simulink model "pmsm_mpc_ekf"  (R2022a)
settings: Solver=ode23tb  StartTime=0.0  StopTime=simlength  FixedStep=tsample  MaxStep=ts
values from neighbouring files (symbols this model uses):
  ki_w = 1    [init.m]    (also in init_2022_05_28.m)
  kp_w = 2    [init.m]    (also in init_2022_05_28.m)
  simlength = 60    [init.m]    (also in init_2022_05_28.m)
  tcontrol = 1/fPWM_INV/6    (= 2.08333333333e-05)    [init.m]    (also in init_2022_05_28.m)
  ts = tcontrol    (= 2.08333333333e-05)    [init.m]    (also in init_2022_05_28.m)
undefined symbols (not defined in the file or in its folder): A1_tilde, A2_tilde, A3_tilde, A4_tilde, Adrso, b, b_brake, Bd, C, Crso, ibez, Jm, Lalpha, Lbeta, Ldrso, omega_bez, omega_m_bez, omega_m_sim, psi_m, Qkalman, Rkalman, Rs, tau_bez, Vdc
libraries: nesl_utility x14, fl_lib x7, pmsm_alphabeta_lib x1
settings Model: SimulationMode=accelerator  Creator=dbagn  LastModifiedBy=dabagnara
settings SolverCC: NumberNewtonIterations=3  ZeroCrossControl=DisableAll  AlgebraicLoopSolver=TrustRegion  SolverResetMethod=Robust
settings DataIOCC: ReturnWorkspaceOutputs=off
settings DebuggingCC: UnconnectedInputMsg=warning  UnconnectedOutputMsg=warning  UnconnectedLineMsg=warning  SFMachineParentedDataDiag=warning
settings RTWCC: DLArmComputeVersion=19.05

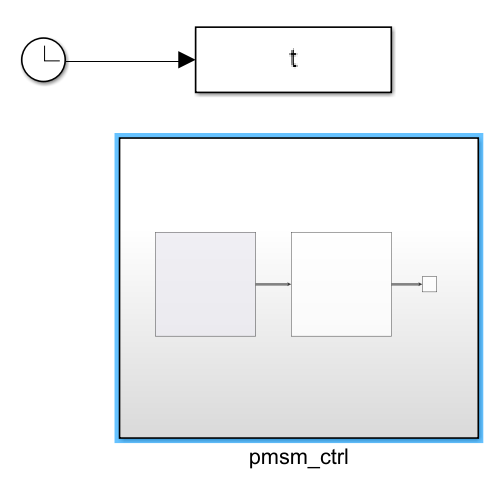
[thumbnail: Simulink's stored preview of the top-level diagram]
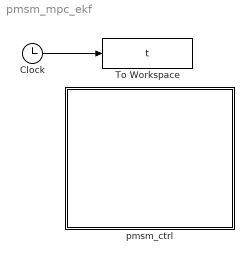
== system pmsm_mpc_ekf ==
  Clock : Clock
  To Workspace : ToWorkspace  VariableName=t  SampleTime=ts
      settings: MaxDataPoints=Nc
  pmsm_ctrl : Subsystem
  wires:
  Clock/1 -> To Workspace/1

== system pmsm_mpc_ekf/pmsm_ctrl ==
  pmsm : Subsystem
  pmsm_control : Subsystem
  pmsm_data : Scope
  wires:
  pmsm_control/1(ualphabeta) -> pmsm/1(u_alphabeta)
  pmsm/1(pmsm_data) -> pmsm_data/1

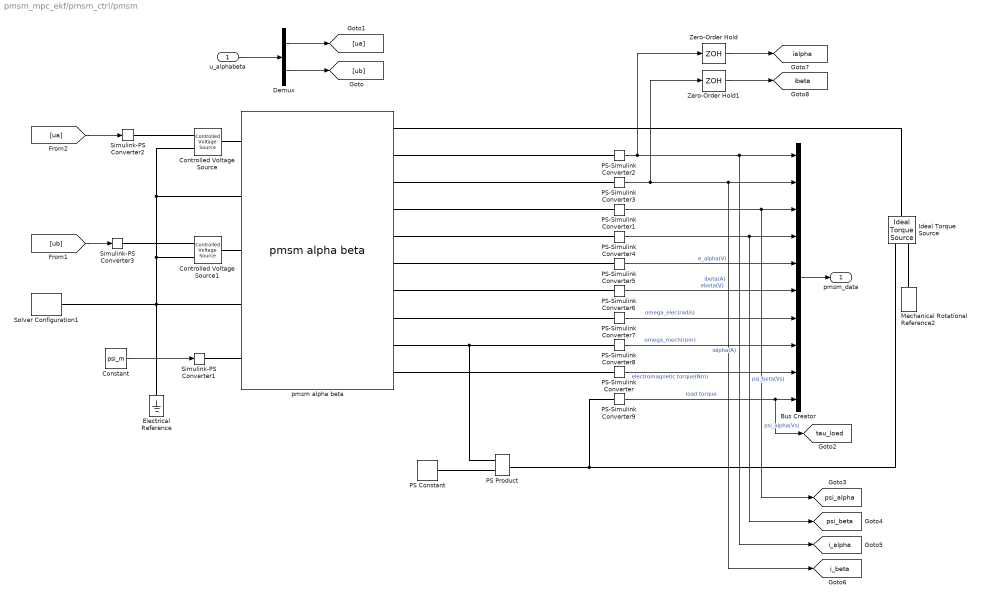
== system pmsm_mpc_ekf/pmsm_ctrl/pmsm ==
  u_alphabeta : Inport
  Bus Creator : BusCreator  Inputs=10
  Constant : Constant  Value=psi_m
  Controlled Voltage Source : fl_lib/Electrical/Electrical Sources/Controlled Voltage Source
      settings: SourceProductBaseCode=PW,SS,VE
  Controlled Voltage Source1 : fl_lib/Electrical/Electrical Sources/Controlled Voltage Source
      settings: SourceProductBaseCode=PW,SS,VE
  Demux : Demux  Outputs=2
  Electrical Reference : fl_lib/Electrical/Electrical Elements/Electrical Reference
      settings: SourceProductBaseCode=PW,SS,VE
  Ideal Torque Source : fl_lib/Mechanical/Mechanical Sources/Ideal Torque Source
      settings: SourceProductBaseCode=PW,SS,VE
  Mechanical Rotational Reference2 : fl_lib/Mechanical/Rotational Elements/Mechanical Rotational Reference
      settings: SourceProductBaseCode=PW,SS,VE
  PS Constant : fl_lib/Physical Signals/Sources/PS Constant  constant=-b_brake N*m/(rad/s)
      settings: SourceProductBaseCode=PW,SS,VE
  PS Product : fl_lib/Physical Signals/Functions/PS Product
      settings: SourceProductBaseCode=PW,SS,VE
  PS-Simulink Converter : nesl_utility/PS-Simulink Converter  PhysicalDomain=network_engine_domain  SubClassName=ps_output  LeftPortType=input  RightPortType=output  PseudoPeriodic=off  Frequencies=[]  VectorFormat=1-D array  Unit=N*m  AffineConversion=on
      settings: SourceProductBaseCode=SS,PW,VE
  PS-Simulink Converter1 : nesl_utility/PS-Simulink Converter  PhysicalDomain=network_engine_domain  SubClassName=ps_output  LeftPortType=input  RightPortType=output  PseudoPeriodic=off  Frequencies=[]  VectorFormat=1-D array  Unit=V*s  AffineConversion=on
      settings: SourceProductBaseCode=SS,PW,VE
  PS-Simulink Converter2 : nesl_utility/PS-Simulink Converter  PhysicalDomain=network_engine_domain  SubClassName=ps_output  LeftPortType=input  RightPortType=output  PseudoPeriodic=off  Frequencies=[]  VectorFormat=1-D array  Unit=A  AffineConversion=on
      settings: SourceProductBaseCode=SS,PW,VE
  PS-Simulink Converter3 : nesl_utility/PS-Simulink Converter  PhysicalDomain=network_engine_domain  SubClassName=ps_output  LeftPortType=input  RightPortType=output  PseudoPeriodic=off  Frequencies=[]  VectorFormat=1-D array  Unit=A  AffineConversion=on
      settings: SourceProductBaseCode=SS,PW,VE
  PS-Simulink Converter4 : nesl_utility/PS-Simulink Converter  PhysicalDomain=network_engine_domain  SubClassName=ps_output  LeftPortType=input  RightPortType=output  PseudoPeriodic=off  Frequencies=[]  VectorFormat=1-D array  Unit=V*s  AffineConversion=on
      settings: SourceProductBaseCode=SS,PW,VE
  PS-Simulink Converter5 : nesl_utility/PS-Simulink Converter  PhysicalDomain=network_engine_domain  SubClassName=ps_output  LeftPortType=input  RightPortType=output  PseudoPeriodic=off  Frequencies=[]  VectorFormat=1-D array  Unit=V  AffineConversion=on
      settings: SourceProductBaseCode=SS,PW,VE
  PS-Simulink Converter6 : nesl_utility/PS-Simulink Converter  PhysicalDomain=network_engine_domain  SubClassName=ps_output  LeftPortType=input  RightPortType=output  PseudoPeriodic=off  Frequencies=[]  VectorFormat=1-D array  Unit=V  AffineConversion=on
      settings: SourceProductBaseCode=SS,PW,VE
  PS-Simulink Converter7 : nesl_utility/PS-Simulink Converter  PhysicalDomain=network_engine_domain  SubClassName=ps_output  LeftPortType=input  RightPortType=output  PseudoPeriodic=off  Frequencies=[]  VectorFormat=1-D array  Unit=rad/s  AffineConversion=on
      settings: SourceProductBaseCode=SS,PW,VE
  PS-Simulink Converter8 : nesl_utility/PS-Simulink Converter  PhysicalDomain=network_engine_domain  SubClassName=ps_output  LeftPortType=input  RightPortType=output  PseudoPeriodic=off  Frequencies=[]  VectorFormat=1-D array  Unit=rpm  AffineConversion=on
      settings: SourceProductBaseCode=SS,PW,VE
  PS-Simulink Converter9 : nesl_utility/PS-Simulink Converter  PhysicalDomain=network_engine_domain  SubClassName=ps_output  LeftPortType=input  RightPortType=output  PseudoPeriodic=off  Frequencies=[]  VectorFormat=1-D array  Unit=N*m  AffineConversion=on
      settings: SourceProductBaseCode=SS,PW,VE
  Simulink-PS Converter1 : nesl_utility/Simulink-PS Converter  PhysicalDomain=network_engine_domain  SubClassName=ps_input  LeftPortType=input  RightPortType=output  PseudoPeriodic=off  Frequencies=[]  NoiseDistribution=none  NoiseParameters=[]  Unit=V*s  AffineConversion=off  FilteringAndDerivatives=provide  SimscapeFilterOrder=1  InputFilterTimeConstant=0.001  UdotUserProvided=0
      settings: SourceProductBaseCode=SS,PW,VE
  Simulink-PS Converter2 : nesl_utility/Simulink-PS Converter  PhysicalDomain=network_engine_domain  SubClassName=ps_input  LeftPortType=input  RightPortType=output  PseudoPeriodic=off  Frequencies=[]  NoiseDistribution=none  NoiseParameters=[]  Unit=1  AffineConversion=off  FilteringAndDerivatives=provide  SimscapeFilterOrder=1  InputFilterTimeConstant=0.001  UdotUserProvided=0
      settings: SourceProductBaseCode=SS,PW,VE
  Simulink-PS Converter3 : nesl_utility/Simulink-PS Converter  PhysicalDomain=network_engine_domain  SubClassName=ps_input  LeftPortType=input  RightPortType=output  PseudoPeriodic=off  Frequencies=[]  NoiseDistribution=none  NoiseParameters=[]  Unit=1  AffineConversion=off  FilteringAndDerivatives=provide  SimscapeFilterOrder=1  InputFilterTimeConstant=0.001  UdotUserProvided=0
      settings: SourceProductBaseCode=SS,PW,VE
  Solver Configuration1 : nesl_utility/Solver Configuration  PhysicalDomain=network_engine_domain  SubClassName=solver  LeftPortType=input  RightPortType=generic  Tones=[]  Harmonics=[]  SimulateNoise=off  Profile=off  UseLocalSampling=off  EnableSwitchedLinearOptims=on  FrequencyDomain=off  UseCCode=off  RelTol=0.001  AbsTol=1e-06  MinStep=1e-09  ToWorkspace=off  RevertToSquareIcSolve=off  NumHomotopyIterations=100  PhasorMode=off  PhasorModeNumHarmonics=1  IndexReductionMethod=DerivativeReplacement  DoDC=on  ResidualTolerance=1e-09  UseLocalSolver=on  LocalSolverChoice=NE_TRAPEZOIDAL_ADVANCER  LocalSolverSampleTime=ts  DoFixedCost=on  MaxNonlinIter=3  MaxModeIter=2  ComputeImpulses=off  ImpulseIterations=2  LinearAlgebra=auto  LinearAlgebraNumThread=0  EquationFormulation=NE_TIME_EF  DelaysMemoryBudget=1024*4  AutomaticFiltering=on  FilteringTimeConstant=ts  PartitionStorageMethod=AS_NEEDED  PartitionMemoryBudget=1024  PartitionMethod=ROBUST
      settings: SourceProductBaseCode=SS,PW,VE
  Zero-Order Hold : ZeroOrderHold  SampleTime=tcontrol
  Zero-Order Hold1 : ZeroOrderHold  SampleTime=tcontrol
  pmsm alpha beta : pmsm_alphabeta_lib/pmsm alpha beta  number_poles=number_poles  Lalpha=Lalpha H  Lbeta=Lbeta H  Rs=Rs Ohm  J=Jm kg*m^2  b=b N*m/(rad/s)  theta_specify=off  theta_priority=None  theta=0 rad  theta_nominal_specify=off  theta_nominal_unit=rad  theta_nominal_value=1  omega_specify=off  omega_priority=None  omega=0 rad/s  omega_nominal_specify=off  omega_nominal_unit=rad/s  omega_nominal_value=1  omega_m_specify=off  omega_m_priority=None  omega_m=0 rad/s  omega_m_nominal_specify=off  omega_m_nominal_unit=rad/s  omega_m_nominal_value=1  ialpha_specify=on  ialpha_priority=High  ialpha=0 A  ialpha_nominal_specify=off  ialpha_nominal_unit=A  ialpha_nominal_value=1  ibeta_specify=on  ibeta_priority=High  ibeta=0 A  ibeta_nominal_specify=off  ibeta_nominal_unit=A  ibeta_nominal_value=1  psi_alpha_specify=off  psi_alpha_priority=None  psi_alpha=0 V*s  psi_alpha_nominal_specify=off  psi_alpha_nominal_unit=V*s  psi_alpha_nominal_value=1  psi_beta_specify=off  psi_beta_priority=High  psi_beta=0.0 V*s  psi_beta_nominal_specify=off  psi_beta_nominal_unit=V*s  psi_beta_nominal_value=1  ualpha_specify=off  ualpha_priority=None  ualpha=0 V  ualpha_nominal_specify=off  ualpha_nominal_unit=V  ualpha_nominal_value=1  ubeta_specify=off  ubeta_priority=None  ubeta=0 V  ubeta_nominal_specify=off  ubeta_nominal_unit=V  ubeta_nominal_value=1  tau_load_specify=off  tau_load_priority=None  tau_load=0 N*m  tau_load_nominal_specify=off  tau_load_nominal_unit=N*m  tau_load_nominal_value=1
      settings: InternalSimscapePortConfiguration="{\"Bottom\":[],\"Left\":[{\"id\":\"u_alpha_p\",\"label\":\"_u_alpha+_\",\"type\":\"foundation.electrical.electrical\"},{\"id\":\"u_alpha_n\",\"label\":\"_u_alpha-_\",\"type\":\"foundation.electrical.electrical\"},{\"id\":\"u_beta_p\",\"label\":\"_u_beta+_\",\"type\":\"foundation.electrical.electrical\"},{\"id\":\"u_beta_n\",\"label\":\"_u_beta-_\",\"type\":\"foundation.electrical.electrical\"},{\"id\":\"psi_m\",\"label\":\"_psi_m_\",\"type\":\"input\"}],\"Right\":[{\"id\":\"s\",\"label\":\"_s_\",\"type\":\"foundation.mechanical.rotational.rotational\"},{\"id\":\"i_alpha_out\",\"label\":\"_i_alpha_\",\"type\":\"output\"},{\"id\":\"i_beta_out\",\"label\":\"_i_beta_\",\"type\":\"output\"},{\"id\":\"psi_alpha_out\",\"label\":\"_psi_alpha_\",\"type\":\"output\"},{\"id\":\"psi_beta_out\",\"label\":\"_psi_beta_\",\"type\":\"output\"},{\"id\":\"e_alpha_out\",\"label\":\"_e_alpha_\",\"type\":\"output\"},{\"id\":\"e_beta_out\",\"label\":\"_e_beta_\",\"type\":\"output\"},{\"id\":\"omega_elec_out\",\"label\":\"_omega_elec_\",\"type\":\"output\"},{\"id\":\"omega_mech_out\",\"label\":\"_omega_mech_\",\"type\":\"output\"},{\"id\":\"torque_e_out\",\"label\":\"_torque_e_\",\"type\":\"output\"}],\"Top\":[]}"
  pmsm_data : Outport
  tag scope: i_alpha=global, i_beta=global, ialpha=global, ibeta=global, psi_alpha=global, psi_beta=global, tau_load=global
  wires:
  [ua] -> Simulink-PS Converter2/1
  [ub] -> Simulink-PS Converter3/1
  u_alphabeta/1 -> Demux/1
  Demux/1 -> [ua]
  Demux/2 -> [ub]
  Zero-Order Hold/1 -> [ialpha]
  Zero-Order Hold1/1 -> [ibeta]
  PS-Simulink Converter2/1 -> [i_alpha], Bus Creator/1, Zero-Order Hold/1  "ialpha(A)"
  PS-Simulink Converter3/1 -> [i_beta], Bus Creator/2, Zero-Order Hold1/1  "ibeta(A)"
  PS-Simulink Converter1/1 -> [psi_alpha], Bus Creator/3  "psi_alpha(Vs)"
  PS-Simulink Converter4/1 -> Bus Creator/4, [psi_beta]  "psi_beta(Vs)"
  PS-Simulink Converter5/1 -> Bus Creator/5  "e_alpha(V)"
  PS-Simulink Converter6/1 -> Bus Creator/6  "ebeta(V)"
  PS-Simulink Converter7/1 -> Bus Creator/7  "omega_elec(rad/s)"
  PS-Simulink Converter8/1 -> Bus Creator/8  "omega_mech(rpm)"
  PS-Simulink Converter/1 -> Bus Creator/9  "electromagnetic torque(Nm)"
  PS-Simulink Converter9/1 -> Bus Creator/10, [tau_load]  "load torque"
  Bus Creator/1 -> pmsm_data/1
  Constant/1 -> Simulink-PS Converter1/1
  connections:
  Controlled Voltage Source/RConn1 -- Simulink-PS Converter2/RConn1
  pmsm alpha beta/LConn1 -- Controlled Voltage Source/LConn1
  Simulink-PS Converter3/RConn1 -- Controlled Voltage Source1/RConn1
  pmsm alpha beta/LConn3 -- Controlled Voltage Source1/LConn1
  Controlled Voltage Source/RConn2 -- Controlled Voltage Source1/RConn2 -- pmsm alpha beta/LConn4 -- Electrical Reference/LConn1 -- Solver Configuration1/RConn1 -- pmsm alpha beta/LConn2
  pmsm alpha beta/RConn2 -- PS-Simulink Converter2/LConn1
  pmsm alpha beta/RConn3 -- PS-Simulink Converter3/LConn1
  PS-Simulink Converter4/LConn1 -- pmsm alpha beta/RConn5
  PS-Simulink Converter1/LConn1 -- pmsm alpha beta/RConn4
  PS-Simulink Converter5/LConn1 -- pmsm alpha beta/RConn6
  pmsm alpha beta/RConn7 -- PS-Simulink Converter6/LConn1
  Mechanical Rotational Reference2/LConn1 -- Ideal Torque Source/RConn2
  pmsm alpha beta/RConn1 -- Ideal Torque Source/LConn1
  pmsm alpha beta/RConn9 -- PS-Simulink Converter8/LConn1 -- PS Product/LConn1
  pmsm alpha beta/RConn10 -- PS-Simulink Converter/LConn1
  PS Constant/RConn1 -- PS Product/LConn2
  PS Product/RConn1 -- Ideal Torque Source/RConn1 -- PS-Simulink Converter9/LConn1
  pmsm alpha beta/RConn8 -- PS-Simulink Converter7/LConn1
  Simulink-PS Converter1/RConn1 -- pmsm alpha beta/LConn5

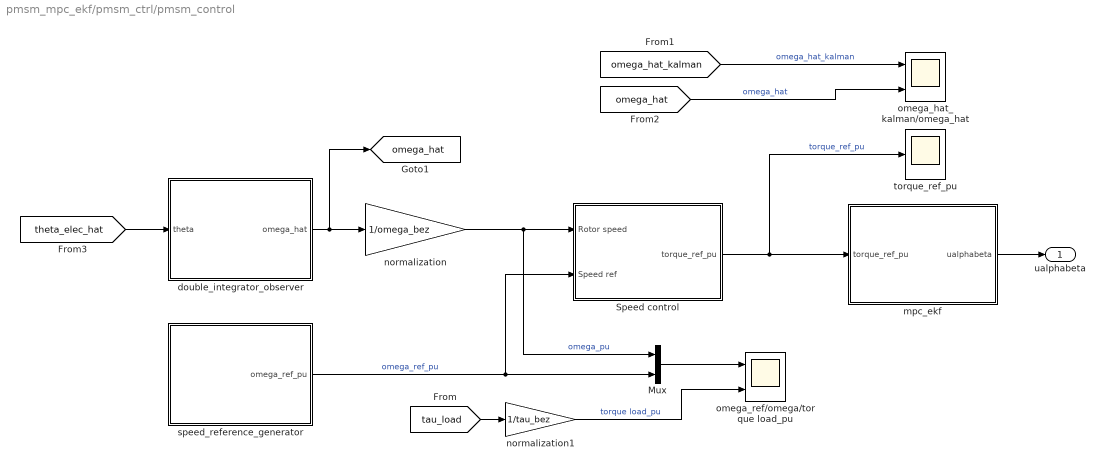
== system pmsm_mpc_ekf/pmsm_ctrl/pmsm_control ==
  Mux : Mux  Inputs=2
  Speed control : Subsystem
  double_integrator_observer : Subsystem
  mpc_ekf : Subsystem
  normalization : Gain  Gain=1/omega_bez
  normalization1 : Gain  Gain=1/tau_bez
  omega_hat_kalman/omega_hat : Scope  NumInputPorts=2
  omega_ref/omega/torque load_pu : Scope  NumInputPorts=2
  speed_reference_generator : Subsystem
  torque_ref_pu : Scope
  ualphabeta : Outport  VectorParamsAs1DForOutWhenUnconnected=off
  tag scope: omega_hat=global
  wires:
  mpc_ekf/1(ualphabeta) -> ualphabeta/1
  normalization/1 -> Mux/1, Speed control/1(Rotor speed)  "omega_pu"
  [theta_elec_hat] -> double_integrator_observer/1(theta)
  Speed control/1(torque_ref_pu) -> torque_ref_pu/1, mpc_ekf/1(torque_ref_pu)  "torque_ref_pu"
  speed_reference_generator/1(omega_ref_pu) -> Speed control/2(Speed ref), Mux/2  "omega_ref_pu"
  Mux/1 -> omega_ref/omega/torque load_pu/1
  [tau_load] -> normalization1/1
  normalization1/1 -> omega_ref/omega/torque load_pu/2  "torque load_pu"
  double_integrator_observer/1(omega_hat) -> [omega_hat], normalization/1
  [omega_hat_kalman] -> omega_hat_kalman/omega_hat/1  "omega_hat_kalman"
  [omega_hat] -> omega_hat_kalman/omega_hat/2  "omega_hat"

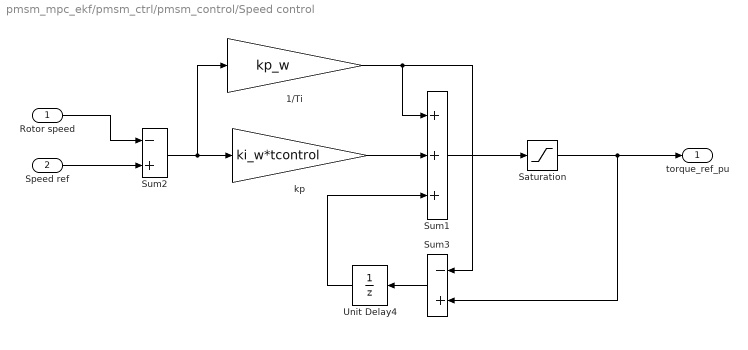
== system pmsm_mpc_ekf/pmsm_ctrl/pmsm_control/Speed control ==
  Rotor speed : Inport
  Speed ref : Inport  Port=2
  1/Ti : Gain  Gain=kp_w  SaturateOnIntegerOverflow=on  OutDataTypeStr=Inherit: Same as input  ParamDataTypeStr=Inherit: Same as input
  Saturation : Saturate  UpperLimit=1.5  LowerLimit=-1.5
  Sum1 : Sum  Inputs=+++  SaturateOnIntegerOverflow=on
  Sum2 : Sum  Inputs=-+  SaturateOnIntegerOverflow=on
  Sum3 : Sum  Inputs=-+  SaturateOnIntegerOverflow=on
  Unit Delay4 : UnitDelay  SampleTime=tcontrol  HasFrameUpgradeWarning=on
  kp : Gain  Gain=ki_w*tcontrol  SaturateOnIntegerOverflow=on  OutDataTypeStr=Inherit: Same as input  ParamDataTypeStr=Inherit: Same as input
  torque_ref_pu : Outport
  wires:
  1/Ti/1 -> Sum1/1, Sum3/1
  kp/1 -> Sum1/2
  Sum3/1 -> Unit Delay4/1
  Unit Delay4/1 -> Sum1/3
  Speed ref/1 -> Sum2/2
  Rotor speed/1 -> Sum2/1
  Sum2/1 -> kp/1, 1/Ti/1
  Saturation/1 -> torque_ref_pu/1, Sum3/2
  Sum1/1 -> Saturation/1

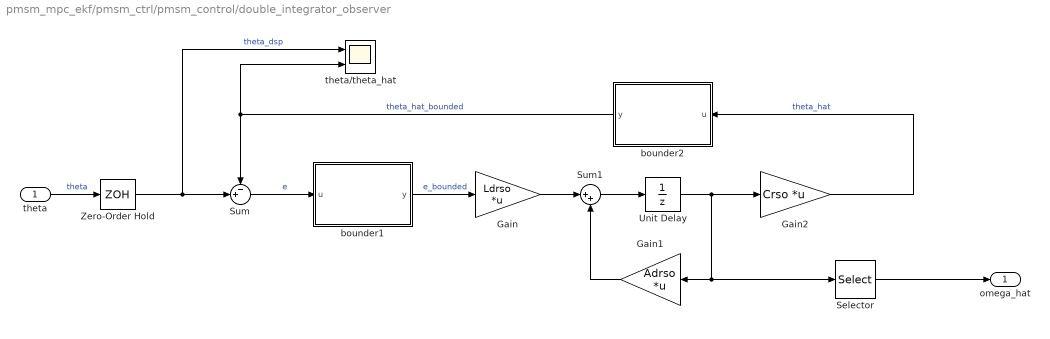
== system pmsm_mpc_ekf/pmsm_ctrl/pmsm_control/double_integrator_observer ==
  theta : Inport
  Gain : Gain  Gain=Ldrso  Multiplication=Matrix(K*u)
  Gain1 : Gain  Gain=Adrso  Multiplication=Matrix(K*u)
  Gain2 : Gain  Gain=Crso  Multiplication=Matrix(K*u)
  Selector : Selector  InputPortWidth=2  IndexOptions=Index vector (dialog)  Indices=2  OutputSizes=1
  Sum : Sum  Inputs=-+|
  Sum1 : Sum  Inputs=|++
  Unit Delay : UnitDelay  SampleTime=tcontrol  HasFrameUpgradeWarning=on
  Zero-Order Hold : ZeroOrderHold  SampleTime=tcontrol
  bounder1 : MATLAB Function  TreatAsAtomicUnit=on  SystemSampleTime=tcontrol
  bounder2 : MATLAB Function  TreatAsAtomicUnit=on  SystemSampleTime=tcontrol
  theta/theta_hat : Scope  NumInputPorts=2
  omega_hat : Outport
  wires:
  Gain/1 -> Sum1/1
  Selector/1 -> omega_hat/1
  Gain2/1 -> bounder2/1(u)  "theta_hat"
  Gain1/1 -> Sum1/2
  Sum1/1 -> Unit Delay/1
  Sum/1 -> bounder1/1(u)  "e"
  Unit Delay/1 -> Gain1/1, Selector/1, Gain2/1
  theta/1 -> Zero-Order Hold/1  "theta"
  Zero-Order Hold/1 -> theta/theta_hat/1, Sum/2  "theta_dsp"
  bounder1/1(y) -> Gain/1  "e_bounded"
  bounder2/1(y) -> theta/theta_hat/2, Sum/1  "theta_hat_bounded"

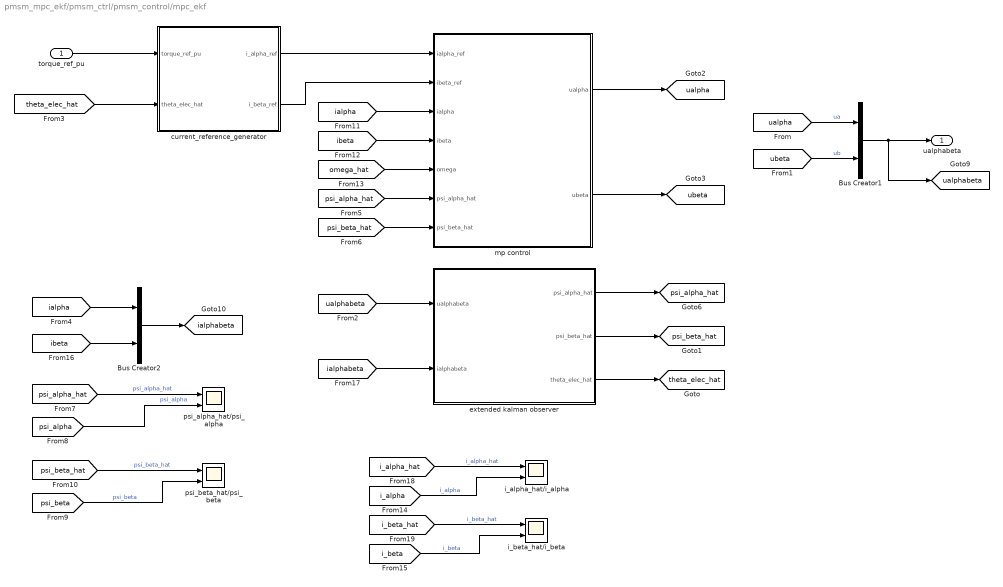
== system pmsm_mpc_ekf/pmsm_ctrl/pmsm_control/mpc_ekf ==
  torque_ref_pu : Inport
  Bus Creator1 : BusCreator  Inputs=2
  Bus Creator2 : BusCreator  Inputs=2
  current_reference_generator : Subsystem
  extended kalman observer : Subsystem
  i_alpha_hat/i_alpha : Scope  NumInputPorts=2
  i_beta_hat/i_beta : Scope  NumInputPorts=2
  mp control : Subsystem
  psi_alpha_hat/psi_alpha : Scope  NumInputPorts=2
  psi_beta_hat/psi_beta : Scope  NumInputPorts=2
  ualphabeta : Outport  VectorParamsAs1DForOutWhenUnconnected=off
  tag scope: ialphabeta=global, psi_alpha_hat=global, psi_beta_hat=global, theta_elec_hat=global, ualpha=global, ualphabeta=global, ubeta=global
  wires:
  [ubeta] -> Bus Creator1/2  "ub"
  [ualpha] -> Bus Creator1/1  "ua"
  Bus Creator1/1 -> [ualphabeta], ualphabeta/1
  torque_ref_pu/1 -> current_reference_generator/1(torque_ref_pu)
  mp control/2(ubeta) -> [ubeta]
  mp control/1(ualpha) -> [ualpha]
  extended kalman observer/1(psi_alpha_hat) -> [psi_alpha_hat]
  extended kalman observer/2(psi_beta_hat) -> [psi_beta_hat]
  [psi_alpha_hat] -> mp control/6(psi_alpha_hat)
  [psi_beta_hat] -> mp control/7(psi_beta_hat)
  [ialpha] -> mp control/3(ialpha)
  [ibeta] -> mp control/4(ibeta)
  [omega_hat] -> mp control/5(omega)
  current_reference_generator/1(i_alpha_ref) -> mp control/1(ialpha_ref)
  current_reference_generator/2(i_beta_ref) -> mp control/2(ibeta_ref)
  [ualphabeta] -> extended kalman observer/1(ualphabeta)
  [ialpha] -> Bus Creator2/1
  [ibeta] -> Bus Creator2/2
  Bus Creator2/1 -> [ialphabeta]
  [ialphabeta] -> extended kalman observer/2(ialphabeta)
  [theta_elec_hat] -> current_reference_generator/2(theta_elec_hat)
  extended kalman observer/3(theta_elec_hat) -> [theta_elec_hat]
  [psi_alpha_hat] -> psi_alpha_hat/psi_alpha/1  "psi_alpha_hat"
  [psi_alpha] -> psi_alpha_hat/psi_alpha/2  "psi_alpha"
  [psi_beta_hat] -> psi_beta_hat/psi_beta/1  "psi_beta_hat"
  [psi_beta] -> psi_beta_hat/psi_beta/2  "psi_beta"
  [i_alpha_hat] -> i_alpha_hat/i_alpha/1  "i_alpha_hat"
  [i_alpha] -> i_alpha_hat/i_alpha/2  "i_alpha"
  [i_beta_hat] -> i_beta_hat/i_beta/1  "i_beta_hat"
  [i_beta] -> i_beta_hat/i_beta/2  "i_beta"

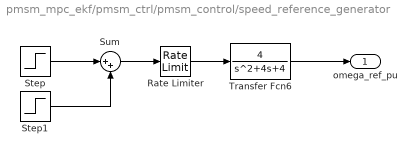
== system pmsm_mpc_ekf/pmsm_ctrl/pmsm_control/speed_reference_generator ==
  Rate Limiter : RateLimiter  RisingSlewLimit=0.25  FallingSlewLimit=-0.25  SampleTimeMode=inherited
  Step : Step  Time=simlength/20  After=omega_m_sim/omega_m_bez  SampleTime=0
  Step1 : Step  Time=simlength/2  After=-2*omega_m_sim/omega_m_bez  SampleTime=0
  Sum : Sum  Inputs=|++
  Transfer Fcn6 : TransferFcn  Numerator=[4]  Denominator=[1 4 4]
  omega_ref_pu : Outport
  wires:
  Rate Limiter/1 -> Transfer Fcn6/1
  Step/1 -> Sum/1
  Transfer Fcn6/1 -> omega_ref_pu/1
  Sum/1 -> Rate Limiter/1
  Step1/1 -> Sum/2

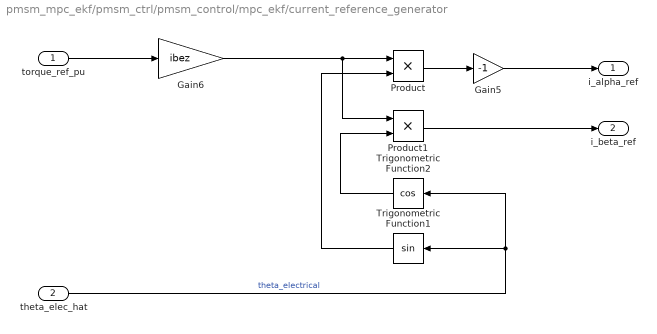
== system pmsm_mpc_ekf/pmsm_ctrl/pmsm_control/mpc_ekf/current_reference_generator ==
  torque_ref_pu : Inport
  theta_elec_hat : Inport  Port=2
  Gain5 : Gain  Gain=-1
  Gain6 : Gain  Gain=ibez
  Product : Product
  Product1 : Product
  Trigonometric Function1 : Trigonometry
  Trigonometric Function2 : Trigonometry  Operator=cos
  i_alpha_ref : Outport
  i_beta_ref : Outport  Port=2
  wires:
  theta_elec_hat/1 -> Trigonometric Function2/1, Trigonometric Function1/1  "theta_electrical"
  Gain6/1 -> Product1/1, Product/1
  Gain5/1 -> i_alpha_ref/1
  Product/1 -> Gain5/1
  Trigonometric Function2/1 -> Product1/2
  Product1/1 -> i_beta_ref/1
  Trigonometric Function1/1 -> Product/2
  torque_ref_pu/1 -> Gain6/1

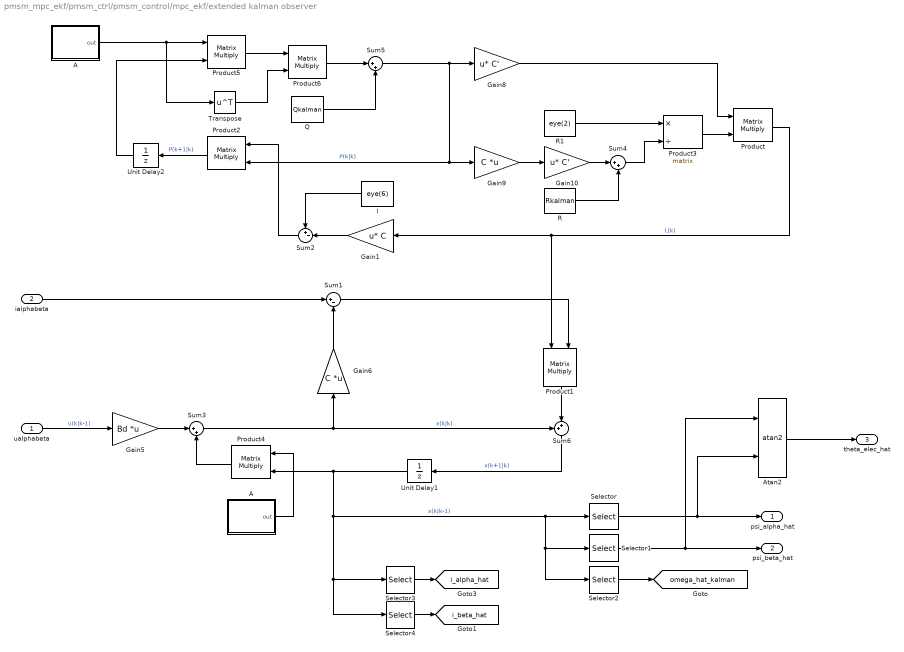
== system pmsm_mpc_ekf/pmsm_ctrl/pmsm_control/mpc_ekf/extended kalman observer ==
  ualphabeta : Inport
  ialphabeta : Inport  Port=2
  A : Subsystem
  "A " : Subsystem
  Atan2 : Trigonometry  Operator=atan2
  Gain1 : Gain  Gain=C  Multiplication=Matrix(u*K)
  Gain10 : Gain  Gain=C'  Multiplication=Matrix(u*K)
  Gain5 : Gain  Gain=Bd  Multiplication=Matrix(K*u)
  Gain6 : Gain  Gain=C  Multiplication=Matrix(K*u)
  Gain8 : Gain  Gain=C'  Multiplication=Matrix(u*K)
  Gain9 : Gain  Gain=C  Multiplication=Matrix(K*u)
  I : Constant  Value=eye(6)
  Product{,1..2,4..6} (6 alike) : Product  Multiplication=Matrix(*)
  Product3 : Product  Inputs=*/  Multiplication=Matrix(*)
  Q : Constant  Value=Qkalman
  R : Constant  Value=Rkalman
  R1 : Constant  Value=eye(2)
  Selector : Selector  InputPortWidth=6  IndexOptions=Index vector (dialog)  Indices=3  OutputSizes=1
  Selector1 : Selector  InputPortWidth=6  IndexOptions=Index vector (dialog)  Indices=4  OutputSizes=1
  Selector2 : Selector  InputPortWidth=6  IndexOptions=Index vector (dialog)  Indices=6  OutputSizes=1
  Selector3 : Selector  InputPortWidth=6  IndexOptions=Index vector (dialog)  Indices=1  OutputSizes=1
  Selector4 : Selector  InputPortWidth=6  IndexOptions=Index vector (dialog)  Indices=2  OutputSizes=1
  Sum1 : Sum  Inputs=|+-
  Sum2 : Sum  Inputs=+-|
  Sum3 : Sum  Inputs=|++
  Sum4 : Sum  Inputs=|++
  Sum5 : Sum  Inputs=|++
  Sum6 : Sum  Inputs=++|
  Transpose : Math  Operator=transpose
  Unit Delay1 : UnitDelay  InitialCondition=[0 0 tcontrol tcontrol 0 0]  SampleTime=tcontrol  HasFrameUpgradeWarning=on
  Unit Delay2 : UnitDelay  SampleTime=tcontrol  HasFrameUpgradeWarning=on
  psi_alpha_hat : Outport
  psi_beta_hat : Outport  Port=2
  theta_elec_hat : Outport  Port=3
  tag scope: i_alpha_hat=global, i_beta_hat=global, omega_hat_kalman=global
  wires:
  Gain5/1 -> Sum3/1
  Product4/1 -> Sum3/2
  Gain6/1 -> Sum1/2
  Sum5/1 -> Product2/2, Gain9/1, Gain8/1  "P(k|k)"
  Product5/1 -> Product6/1
  Product6/1 -> Sum5/1
  Q/1 -> Sum5/2
  Gain9/1 -> Gain10/1
  R/1 -> Sum4/2
  Gain10/1 -> Sum4/1
  Gain8/1 -> Product/1
  Product/1 -> Product1/1, Gain1/1  "L(k)"
  Product2/1 -> Unit Delay2/1  "P(k+1|k)"
  Sum2/1 -> Product2/1
  Unit Delay2/1 -> Product5/2
  Sum6/1 -> Unit Delay1/1  "x(k+1|k)"
  I/1 -> Sum2/1
  Gain1/1 -> Sum2/2
  Sum1/1 -> Product1/2
  ialphabeta/1 -> Sum1/1
  Sum4/1 -> Product3/2
  Product3/1 -> Product/2
  R1/1 -> Product3/1
  ualphabeta/1 -> Gain5/1  "u(k|k-1)"
  Sum3/1 -> Gain6/1, Sum6/1  "x(k|k)"
  Unit Delay1/1 -> Selector4/1, Selector3/1, Selector2/1, Selector1/1, Selector/1, Product4/2  "x(k|k-1)"
  A/1(out) -> Product4/1
  "A "/1(out) -> Transpose/1, Product5/1
  Product1/1 -> Sum6/2
  Selector1/1 -> Atan2/1, psi_beta_hat/1
  Selector/1 -> Atan2/2, psi_alpha_hat/1
  Transpose/1 -> Product6/2
  Selector2/1 -> [omega_hat_kalman]
  Selector3/1 -> [i_alpha_hat]
  Atan2/1 -> theta_elec_hat/1
  Selector4/1 -> [i_beta_hat]

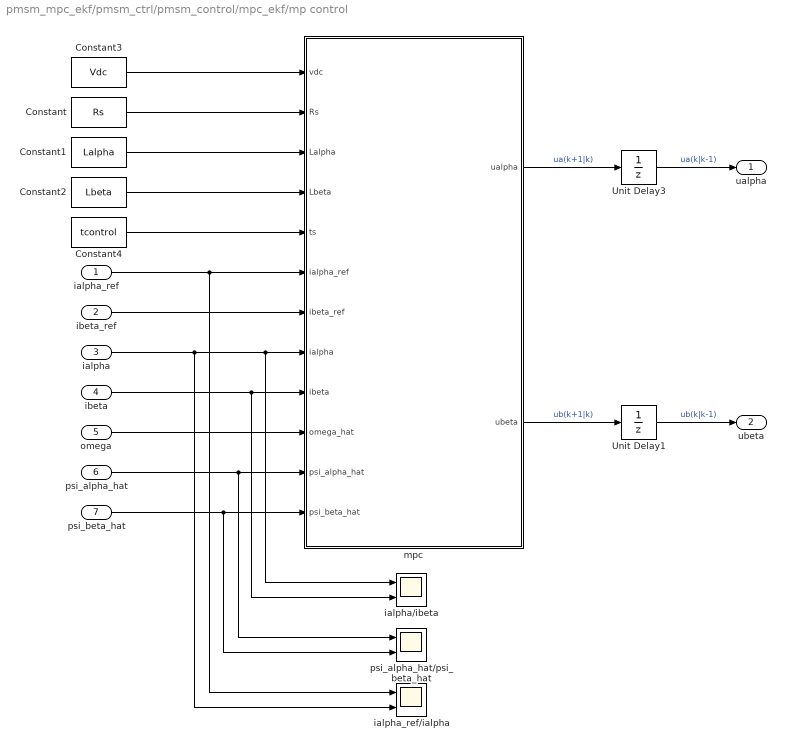
== system pmsm_mpc_ekf/pmsm_ctrl/pmsm_control/mpc_ekf/mp control ==
  ialpha_ref : Inport
  ibeta_ref : Inport  Port=2
  ialpha : Inport  Port=3
  ibeta : Inport  Port=4
  omega : Inport  Port=5
  psi_alpha_hat : Inport  Port=6
  psi_beta_hat : Inport  Port=7
  Constant : Constant  Value=Rs
  Constant1 : Constant  Value=Lalpha
  Constant2 : Constant  Value=Lbeta
  Constant3 : Constant  Value=Vdc
  Constant4 : Constant  Value=tcontrol
  Unit Delay1 : UnitDelay  SampleTime=tcontrol  HasFrameUpgradeWarning=on
  Unit Delay3 : UnitDelay  SampleTime=tcontrol  HasFrameUpgradeWarning=on
  ialpha/ibeta : Scope  NumInputPorts=2
  ialpha_ref/ialpha : Scope  NumInputPorts=2
  mpc : MATLAB Function  TreatAsAtomicUnit=on  SystemSampleTime=tcontrol
  psi_alpha_hat/psi_beta_hat : Scope  NumInputPorts=2
  ualpha : Outport
  ubeta : Outport  Port=2
  wires:
  Constant/1 -> mpc/2(Rs)
  ialpha_ref/1 -> mpc/6(ialpha_ref), ialpha_ref/ialpha/1
  ibeta_ref/1 -> mpc/7(ibeta_ref)
  Constant1/1 -> mpc/3(Lalpha)
  mpc/1(ualpha) -> Unit Delay3/1  "ua(k+1|k)"
  Unit Delay3/1 -> ualpha/1  "ua(k|k-1)"
  Constant3/1 -> mpc/1(vdc)
  Constant4/1 -> mpc/5(ts)
  ialpha/1 -> ialpha/ibeta/1, mpc/8(ialpha), ialpha_ref/ialpha/2
  ibeta/1 -> ialpha/ibeta/2, mpc/9(ibeta)
  Unit Delay1/1 -> ubeta/1  "ub(k|k-1)"
  mpc/2(ubeta) -> Unit Delay1/1  "ub(k+1|k)"
  omega/1 -> mpc/10(omega_hat)
  psi_alpha_hat/1 -> psi_alpha_hat/psi_beta_hat/1, mpc/11(psi_alpha_hat)
  psi_beta_hat/1 -> mpc/12(psi_beta_hat), psi_alpha_hat/psi_beta_hat/2
  Constant2/1 -> mpc/4(Lbeta)

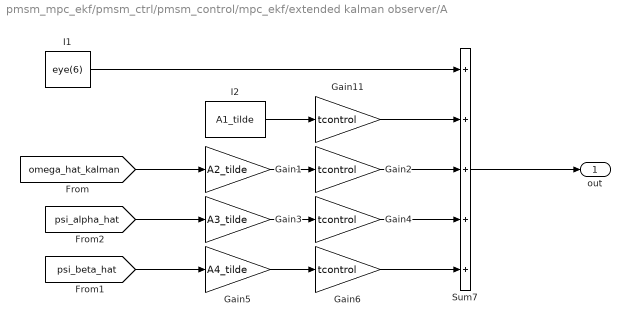
== system pmsm_mpc_ekf/pmsm_ctrl/pmsm_control/mpc_ekf/extended kalman observer/A ==
  Gain1 : Gain  Gain=A2_tilde
  Gain{2,4,6,11} (4 alike) : Gain  Gain=tcontrol
  Gain3 : Gain  Gain=A3_tilde
  Gain5 : Gain  Gain=A4_tilde
  I1 : Constant  Value=eye(6)
  I2 : Constant  Value=A1_tilde
  Sum7 : Sum  Inputs=+++++
  out : Outport
  wires:
  Sum7/1 -> out/1
  I2/1 -> Gain11/1
  I1/1 -> Sum7/1
  Gain11/1 -> Sum7/2
  Gain1/1 -> Gain2/1
  Gain2/1 -> Sum7/3
  Gain3/1 -> Gain4/1
  Gain4/1 -> Sum7/4
  Gain5/1 -> Gain6/1
  Gain6/1 -> Sum7/5
  [omega_hat_kalman] -> Gain1/1
  [psi_alpha_hat] -> Gain3/1
  [psi_beta_hat] -> Gain5/1

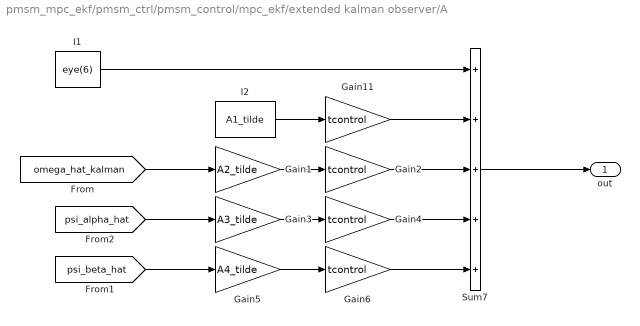
== system pmsm_mpc_ekf/pmsm_ctrl/pmsm_control/mpc_ekf/extended kalman observer/A  ==
  Gain1 : Gain  Gain=A2_tilde
  Gain{2,4,6,11} (4 alike) : Gain  Gain=tcontrol
  Gain3 : Gain  Gain=A3_tilde
  Gain5 : Gain  Gain=A4_tilde
  I1 : Constant  Value=eye(6)
  I2 : Constant  Value=A1_tilde
  Sum7 : Sum  Inputs=+++++
  out : Outport
  wires:
  [psi_beta_hat] -> Gain5/1
  [psi_alpha_hat] -> Gain3/1
  [omega_hat_kalman] -> Gain1/1
  Gain6/1 -> Sum7/5
  Gain5/1 -> Gain6/1
  Gain4/1 -> Sum7/4
  Gain3/1 -> Gain4/1
  Gain2/1 -> Sum7/3
  Gain1/1 -> Gain2/1
  Gain11/1 -> Sum7/2
  I1/1 -> Sum7/1
  I2/1 -> Gain11/1
  Sum7/1 -> out/1

== matlab function pmsm_mpc_ekf/pmsm_ctrl/pmsm_control/double_integrator_observer/bounder1 ==
  data: u input; y output
function y = bounder(u)
    
    u = -pi + mod(u+3*pi,2*pi);
    
    y = u;
end

== matlab function pmsm_mpc_ekf/pmsm_ctrl/pmsm_control/double_integrator_observer/bounder2 ==
  data: u input; y output
function y = bounder(u)
    
    u = -pi + mod(u+3*pi,2*pi);
    
    y = u;
end

== matlab function pmsm_mpc_ekf/pmsm_ctrl/pmsm_control/mpc_ekf/mp control/mpc ==
  data: vdc input; Rs input; Lalpha input; Lbeta input; ts input; ialpha_ref input; ibeta_ref input; ialpha input; ualpha output; ibeta input; omega_hat input; psi_alpha_hat input; psi_beta_hat input; ubeta output
function [ualpha, ubeta]    = mpc(vdc, Rs, Lalpha, Lbeta, ts, ialpha_ref,...
    ibeta_ref, ialpha, ibeta, omega_hat, psi_alpha_hat, psi_beta_hat)

    persistent ualpha_z ubeta_z

    ualpha_1 = 2/3*vdc;
    ubeta_1 = 0;

    ualpha_2 = 2/3*1/2*vdc;
    ubeta_2 = 2/3*sqrt(3)/2*vdc;

    ualpha_3 = -2/3*1/2*vdc;
    ubeta_3 = 2/3*sqrt(3)/2*vdc;

    ualpha_4 = -2/3*vdc;
    ubeta_4 = 0;

    ualpha_5 = -2/3*1/2*vdc;
    ubeta_5 = -2/3*sqrt(3)/2*vdc;

    ualpha_6 = 2/3*1/2*vdc;
    ubeta_6 = -2/3*sqrt(3)/2*vdc;

    ualpha_0 = 0;
    ubeta_0 = 0;

    if isempty(ualpha_z)
        ualpha_z = 0;
        ubeta_z = 0;
    end

    ia_p0 = (1-Rs/Lalpha*ts)*ialpha + omega_hat/Lalpha*psi_beta_hat*ts + ualpha_0*ts/Lalpha;
    ib_p0 = (1-Rs/Lbeta*ts)*ibeta - omega_hat/Lbeta*psi_alpha_hat*ts + ubeta_0*ts/Lbeta;
    
    ia_p1 = (1-Rs/Lalpha*ts)*ialpha + omega_hat/Lalpha*psi_beta_hat*ts + ualpha_1*ts/Lalpha;
    ib_p1 = (1-Rs/Lbeta*ts)*ibeta - omega_hat/Lbeta*psi_alpha_hat*ts + ubeta_1*ts/Lbeta;

    ia_p2 = (1-Rs/Lalpha*ts)*ialpha + omega_hat/Lalpha*psi_beta_hat*ts + ualpha_2*ts/Lalpha;
    ib_p2 = (1-Rs/Lbeta*ts)*ibeta - omega_hat/Lbeta*psi_alpha_hat*ts + ubeta_2*ts/Lbeta;

    ia_p3 = (1-Rs/Lalpha*ts)*ialpha + omega_hat/Lalpha*psi_beta_hat*ts + ualpha_3*ts/Lalpha;
    ib_p3 = (1-Rs/Lbeta*ts)*ibeta - omega_hat/Lbeta*psi_alpha_hat*ts + ubeta_3*ts/Lbeta;

    ia_p4 = (1-Rs/Lalpha*ts)*ialpha + omega_hat/Lalpha*psi_beta_hat*ts + ualpha_4*ts/Lalpha;
    ib_p4 = (1-Rs/Lbeta*ts)*ibeta - omega_hat/Lbeta*psi_alpha_hat*ts + ubeta_4*ts/Lbeta;

    ia_p5 = (1-Rs/Lalpha*ts)*ialpha + omega_hat/Lalpha*psi_beta_hat*ts + ualpha_5*ts/Lalpha;
    ib_p5 = (1-Rs/Lbeta*ts)*ibeta - omega_hat/Lbeta*psi_alpha_hat*ts + ubeta_5*ts/Lbeta;

    ia_p6 = (1-Rs/Lalpha*ts)*ialpha + omega_hat/Lalpha*psi_beta_hat*ts + ualpha_6*ts/Lalpha;
    ib_p6 = (1-Rs/Lbeta*ts)*ibeta - omega_hat/Lbeta*psi_alpha_hat*ts + ubeta_6*ts/Lbeta;
  
    J0 = (ialpha_ref - ia_p0)^2 + (ibeta_ref - ib_p0)^2;
    J1 = (ialpha_ref - ia_p1)^2 + (ibeta_ref - ib_p1)^2;
    J2 = (ialpha_ref - ia_p2)^2 + (ibeta_ref - ib_p2)^2;
    J3 = (ialpha_ref - ia_p3)^2 + (ibeta_ref - ib_p3)^2;
    J4 = (ialpha_ref - ia_p4)^2 + (ibeta_ref - ib_p4)^2;
    J5 = (ialpha_ref - ia_p5)^2 + (ibeta_ref - ib_p5)^2;
    J6 = (ialpha_ref - ia_p6)^2 + (ibeta_ref - ib_p6)^2;
    
    if (ualpha_z == ualpha_0) && (ubeta_z == ubeta_0)
        [m,i] = min([J0, J1, J2, J3, J4, J5, J6]);
        if i == 1
            ualpha = ualpha_0;
            ubeta = ubeta_0;
        elseif i == 2
            ualpha = ualpha_1;
            ubeta = ubeta_1;
        elseif i == 3
            ualpha = ualpha_2;
            ubeta = ubeta_2;
        elseif i == 4
            ualpha = ualpha_3;
            ubeta = ubeta_3;
        elseif i == 5
            ualpha = ualpha_4;
            ubeta = ubeta_4;
        elseif i == 6
            ualpha = ualpha_5;
            ubeta = ubeta_5;
        else
            ualpha = ualpha_6;
            ubeta = ubeta_6;
        end
    elseif (ualpha_z == ualpha_1) && (ubeta_z == ubeta_1)
        [m,i] = min([J0, J1, J2, J6]);
        if i == 1
            ualpha = ualpha_0;
            ubeta = ubeta_0;
        elseif i == 2
            ualpha = ualpha_1;
            ubeta = ubeta_1;
        elseif i == 3
            ualpha = ualpha_2;
            ubeta = ubeta_2;
        else
            ualpha = ualpha_6;
            ubeta = ubeta_6;
        end
    elseif (ualpha_z == ualpha_2) && (ubeta_z == ubeta_2) % vector u2
        [m,i] = min([J0, J1, J2, J3]);
        if i == 1
            ualpha = ualpha_0;
            ubeta = ubeta_0;
        elseif i == 2
            ualpha = ualpha_1;
            ubeta = ubeta_1;
        elseif i == 3
            ualpha = ualpha_2;
            ubeta = ubeta_2;
        else
            ualpha = ualpha_3;
            ubeta = ubeta_3;
        end
    elseif (ualpha_z == ualpha_3) && (ubeta_z == ubeta_3)
        [m,i] = min([J0, J2, J3, J4]);
        if i == 1
            ualpha = ualpha_0;
            ubeta = ubeta_0;
        elseif i == 2
            ualpha = ualpha_2;
            ubeta = ubeta_2;
        elseif i == 3
            ualpha = ualpha_3;
            ubeta = ubeta_3;
        else
            ualpha = ualpha_4;
            ubeta = ubeta_4;
        end
    elseif (ualpha_z == ualpha_4) && (ubeta_z == ubeta_4)
        [m,i] = min([J0, J3, J4, J5]);
        if i == 1
            ualpha = ualpha_0;
            ubeta = ubeta_0;
        elseif i == 2
            ualpha = ualpha_3;
            ubeta = ubeta_3;
        elseif i == 3
            ualpha = ualpha_4;
            ubeta = ubeta_4;
        else
            ualpha = ualpha_5;
            ubeta = ubeta_5;
        end
    elseif (ualpha_z == ualpha_5) && (ubeta_z == ubeta_5) % u5
        [m,i] = min([J0, J4, J5, J6]);
        if i == 1
            ualpha = ualpha_0;
            ubeta = ubeta_0;
        elseif i == 2
            ualpha = ualpha_4;
            ubeta = ubeta_4;
        elseif i == 3
            ualpha = ualpha_5;
            ubeta = ubeta_5;
        else
            ualpha = ualpha_6;
            ubeta = ubeta_6;
        end
    else
        [m,i] = min([J0, J5, J6, J1]);
        if i == 1
            ualpha = ualpha_0;
            ubeta = ubeta_0;
        elseif i == 2
            ualpha = ualpha_5;
            ubeta = ubeta_5;
        elseif i == 3
            ualpha = ualpha_6;
            ubeta = ubeta_6;
        else
            ualpha = ualpha_1;
            ubeta = ubeta_1;
        end
    end
    ualpha_z = ualpha;
    ubeta_z = ubeta;
end
